simulink library "mag_block"  (R2025b)
settings: Solver=VariableStepAuto  StartTime=0.0  StopTime=10.0  RelTol=1e-3
values from neighbouring files (symbols this model uses):
  Mag = evalin('base', 'Mag')    [test_mag_block_visual_compile.m]    (also in test_mag_model.m)
settings Model: Creator=Ashwin  LastModifiedBy=Ashwin

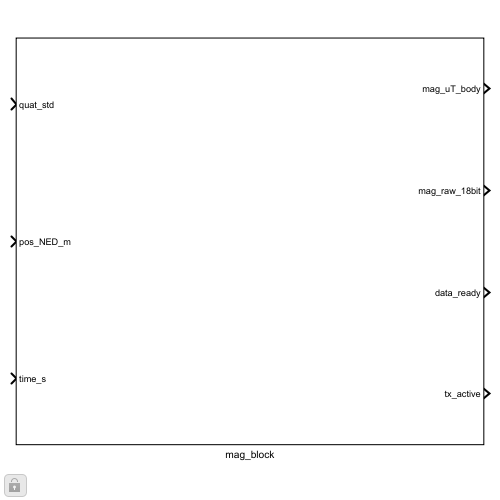
[thumbnail: Simulink's stored preview of the top-level diagram]
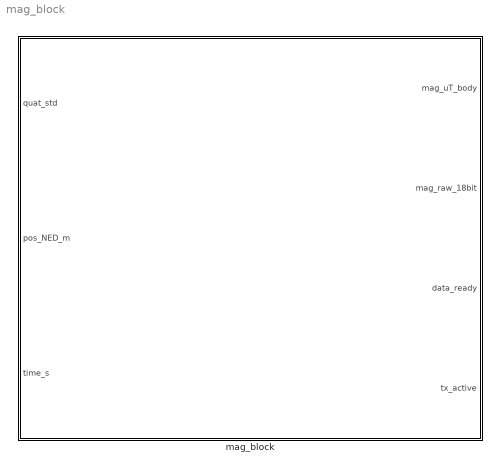
== system mag_block ==
  mag_block : Subsystem

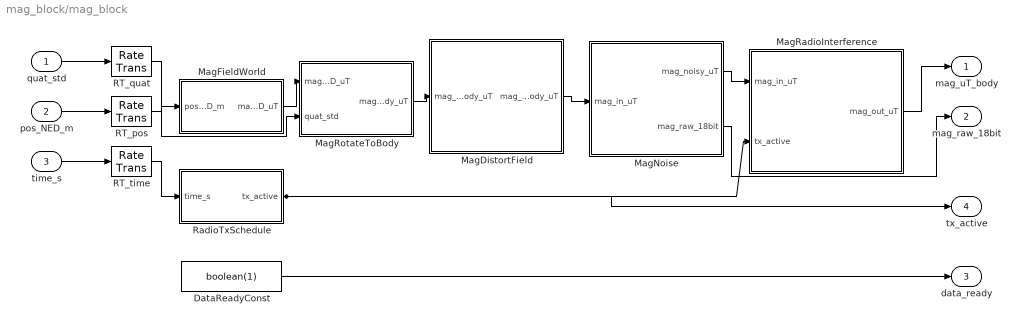
== system mag_block/mag_block ==
  quat_std : Inport  PortDimensions=4
  pos_NED_m : Inport  Port=2  PortDimensions=3
  time_s : Inport  Port=3  PortDimensions=1
  DataReadyConst : Constant  Value=boolean(1)  OutDataTypeStr=boolean  SampleTime=1/Mag.Rate_Hz
  MagDistortField : MATLAB Function  TreatAsAtomicUnit=on
  MagFieldWorld : MATLAB Function  TreatAsAtomicUnit=on
  MagNoise : MATLAB Function  TreatAsAtomicUnit=on
  MagRadioInterference : MATLAB Function  TreatAsAtomicUnit=on
  MagRotateToBody : MATLAB Function  TreatAsAtomicUnit=on
  RT_pos : RateTransition  OutPortSampleTime=1/Mag.Rate_Hz
  RT_quat : RateTransition  OutPortSampleTime=1/Mag.Rate_Hz
  RT_time : RateTransition  OutPortSampleTime=1/Mag.Rate_Hz
  RadioTxSchedule : MATLAB Function  TreatAsAtomicUnit=on
  mag_uT_body : Outport  PortDimensions=3
  mag_raw_18bit : Outport  Port=2  PortDimensions=3
  data_ready : Outport  Port=3  PortDimensions=1
  tx_active : Outport  Port=4  PortDimensions=1
  wires:
  quat_std/1 -> RT_quat/1
  pos_NED_m/1 -> RT_pos/1
  time_s/1 -> RT_time/1
  RT_pos/1 -> MagFieldWorld/1(pos_NED_m)
  MagFieldWorld/1(mag_NED_uT) -> MagRotateToBody/1(mag_NED_uT)
  RT_quat/1 -> MagRotateToBody/2(quat_std)
  MagRotateToBody/1(mag_body_uT) -> MagDistortField/1(mag_clean_body_uT)
  MagDistortField/1(mag_raw_body_uT) -> MagNoise/1(mag_in_uT)
  MagNoise/1(mag_noisy_uT) -> MagRadioInterference/1(mag_in_uT)
  RT_time/1 -> RadioTxSchedule/1(time_s)
  RadioTxSchedule/1(tx_active) -> MagRadioInterference/2(tx_active), tx_active/1
  MagRadioInterference/1(mag_out_uT) -> mag_uT_body/1
  MagNoise/2(mag_raw_18bit) -> mag_raw_18bit/1
  DataReadyConst/1 -> data_ready/1

== matlab function mag_block/MagFieldWorld ==
  data: pos_NED_m input; mag_NED_uT output
function mag_NED_uT = MagFieldWorld(pos_NED_m)
%#codegen
mag_NED_uT = casper_mag_field_world(pos_NED_m);
end

== matlab function mag_block/MagDistortField ==
  data: mag_clean_body_uT input; mag_raw_body_uT output
function mag_raw_body_uT = MagDistortField(mag_clean_body_uT)
%#codegen
coder.extrinsic('evalin');
hard_iron = zeros(3,1);
soft_iron = zeros(3,3);
axis_flip = zeros(3,1);
hard_iron = evalin('base', 'Mag.HardIron_uT');
soft_iron = evalin('base', 'Mag.SoftIron');
axis_flip = evalin('base', 'Mag.AxisFlipSign');
mag_raw_body_uT = casper_mag_distort_field(mag_clean_body_uT, ...
    hard_iron, soft_iron, axis_flip);
end

== matlab function mag_block/MagNoise ==
  data: mag_in_uT input; mag_noisy_uT output; mag_raw_18bit output
function [mag_noisy_uT, mag_raw_18bit] = MagNoise(mag_in_uT)
%#codegen
coder.extrinsic('evalin');
dt_s          = 0.01;
tau_s         = 0.16;
sigma_white   = 0.5;
scale_cpg     = 16384;
offset_counts = 131072;
seed          = uint32(0);
dt_s          = evalin('base', '1/Mag.Rate_Hz');
tau_s         = evalin('base', 'Mag.NoiseTauSec');
sigma_white   = evalin('base', 'Mag.NoiseStd_uT');
scale_cpg     = evalin('base', 'Mag.ScaleCountsPerGauss');
offset_counts = evalin('base', 'Mag.OffsetCounts');
seed          = uint32(evalin('base', 'Sim.Seed + 3'));
mag_noisy_uT  = zeros(3,1);
mag_raw_18bit = uint32(zeros(3,1));
[mag_noisy_uT, mag_raw_18bit] = casper_mag_noise(mag_in_uT, ...
    dt_s, tau_s, sigma_white, scale_cpg, offset_counts, seed);
end

== matlab function mag_block/RadioTxSchedule ==
  data: time_s input; tx_active output
function tx_active = RadioTxSchedule(time_s)
%#codegen
coder.extrinsic('evalin');
tx_period_s  = 0.1;
tx_airtime_s = 0.015;
tx_period_s  = evalin('base', 'Mag.RadioTXPeriod_s');
tx_airtime_s = evalin('base', 'Mag.RadioTXAirtime_s');
tx_active = casper_radio_tx_schedule(time_s, tx_period_s, tx_airtime_s);
end

== matlab function mag_block/MagRadioInterference ==
  data: mag_in_uT input; mag_out_uT output; tx_active input
function mag_out_uT = MagRadioInterference(mag_in_uT, tx_active)
%#codegen
coder.extrinsic('evalin');
interf_active = false;
spike_amp_uT  = 10.0;
seed          = uint32(0);
interf_active = logical(evalin('base', 'Mag.RadioInterfActive'));
spike_amp_uT  = evalin('base', 'Mag.RadioSpikeAmp_uT');
seed          = uint32(evalin('base', 'Sim.Seed + 7'));
mag_out_uT = casper_mag_radio_interference(mag_in_uT, tx_active, ...
    interf_active, spike_amp_uT, seed);
end

== matlab function mag_block/MagRotateToBody ==
  data: mag_NED_uT input; mag_body_uT output; quat_std input
function mag_body_uT = MagRotateToBody(mag_NED_uT, quat_std)
%#codegen
mag_body_uT = casper_mag_rotate_to_body(mag_NED_uT, quat_std);
end
